simulink model "BasicModels"  (R2021b)
settings: Solver=ode45  StartTime=0.0  StopTime=10.0  RelTol=1e-3  EnableMultiTasking=on
settings Model: Creator=User_Admin  LastModifiedBy=User_Admin
settings DataIOCC: LimitDataPoints=on  SaveFormat=Array  SignalLoggingSaveFormat=ModelDataLogs  ReturnWorkspaceOutputs=off
settings OptimizationCC: BooleanDataType=off
settings DebuggingCC: SaveWithParameterizedLinksMsg=none  UnderspecifiedInitializationDetection=Classic  MergeDetectMultiDrivingBlocksExec=none  SignalResolutionControl=TryResolveAllWithWarning  MultiTaskDSMMsg=warning  MultiTaskCondExecSysMsg=none
settings HardwareCC: TargetUnknown=on
settings ModelReferenceCC: PropagateSignalLabelsOutOfModel=off
settings GRTTargetCC: CombineOutputUpdateFcns=off  GRTInterface=on
settings ConfigComp: CovMetricSettings=dw

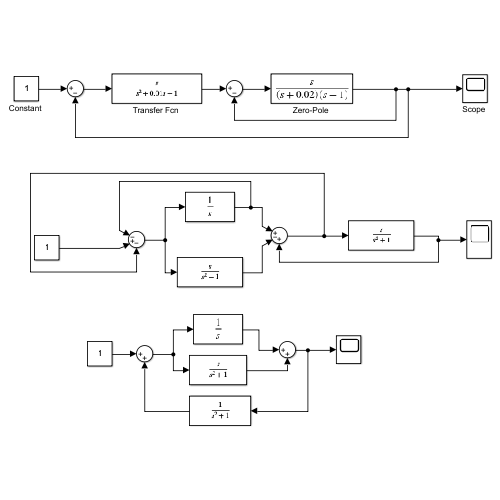
[thumbnail: Simulink's stored preview of the top-level diagram]
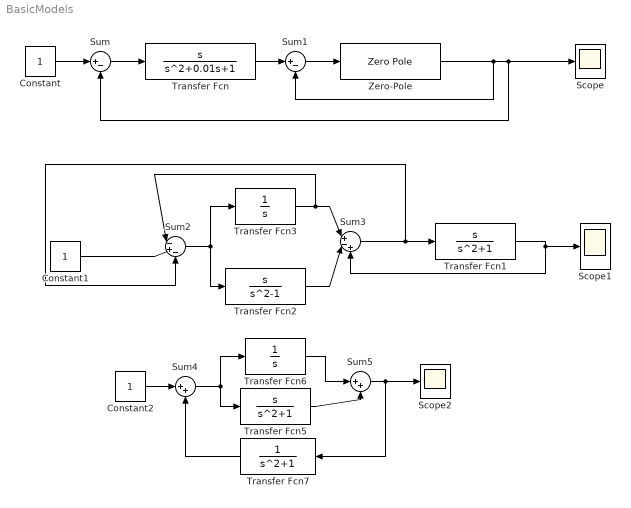
== system BasicModels ==
  "Constant " : Constant
  Constant1 : Constant
  Constant2 : Constant
  "Scope " : Scope
  Scope1 : Scope
  Scope2 : Scope
  Sum : Sum  Inputs=|+-  SaturateOnIntegerOverflow=on
  Sum1 : Sum  Inputs=|+-  SaturateOnIntegerOverflow=on
  Sum2 : Sum  Inputs=|-+-  SaturateOnIntegerOverflow=on
  Sum3 : Sum  Inputs=|+-+  SaturateOnIntegerOverflow=on
  Sum4 : Sum  Inputs=|++  SaturateOnIntegerOverflow=on
  Sum5 : Sum  Inputs=|++  SaturateOnIntegerOverflow=on
  "Transfer Fcn " : TransferFcn  Numerator=[1 0]  Denominator=[1 0.01 1]
  Transfer Fcn1 : TransferFcn  Numerator=[1 0]  Denominator=[1 0 1]
  Transfer Fcn2 : TransferFcn  Numerator=[1 0]  Denominator=[1 0 -1]
  Transfer Fcn3 : TransferFcn  Denominator=[1 0]
  Transfer Fcn5 : TransferFcn  Numerator=[1 0]  Denominator=[1 0 1]
  Transfer Fcn6 : TransferFcn  Denominator=[1 0]
  Transfer Fcn7 : TransferFcn  Numerator=[ 1]  Denominator=[1 0 1]
  "Zero-Pole " : ZeroPole  Zeros=[0]  Poles=[-0.02 -1]
  wires:
  Sum/1 -> "Transfer Fcn "/1
  "Transfer Fcn "/1 -> Sum1/1
  Sum1/1 -> "Zero-Pole "/1
  "Zero-Pole "/1 -> Sum1/2, Sum/2, "Scope "/1
  "Constant "/1 -> Sum/1
  Constant1/1 -> Sum2/2
  Transfer Fcn3/1 -> Sum3/1, Sum2/1
  Sum3/1 -> Transfer Fcn1/1, Sum2/3
  Transfer Fcn2/1 -> Sum3/2
  Transfer Fcn1/1 -> Scope1/1, Sum3/3
  Sum2/1 -> Transfer Fcn2/1, Transfer Fcn3/1
  Constant2/1 -> Sum4/1
  Transfer Fcn6/1 -> Sum5/1
  Sum5/1 -> Scope2/1, Transfer Fcn7/1
  Transfer Fcn5/1 -> Sum5/2
  Sum4/1 -> Transfer Fcn5/1, Transfer Fcn6/1
  Transfer Fcn7/1 -> Sum4/2
